simulink model "modelo_motor_P4_3"  (R2021b)
settings: Solver=VariableStepAuto  StartTime=0.0  StopTime=10.0  RelTol=1e-3
values from neighbouring files (symbols this model uses):
  Kd = Kp*Td    (= 0.032)    [lanza_P4_2.m]
  Ki = Kp/Ti    (= 11.1888111888)    [lanza_P4_2.m]
  Kp = 8    [lanza_P4_2.m]
  Tm = 0.01    [lanza_P4_1.m]    (also in lanza_P4_2.m)
settings Model: Creator=luisb  LastModifiedBy=luisb

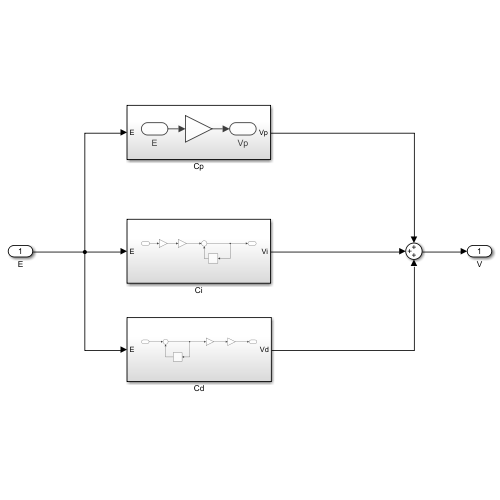
[thumbnail: Simulink's stored preview of the top-level diagram]
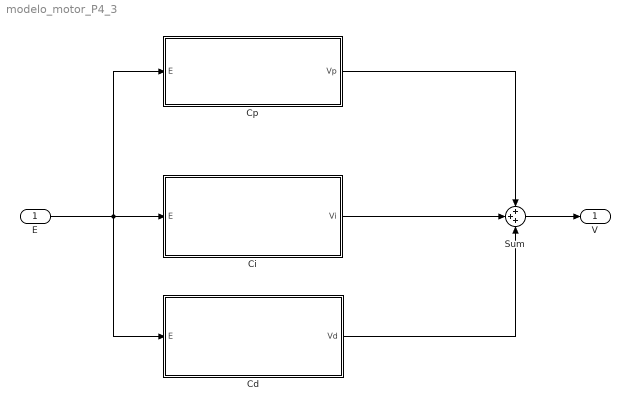
== system modelo_motor_P4_3 ==
  E : Inport
  Cd : Subsystem
  Ci : Subsystem
  Cp : Subsystem
  Sum : Sum  Inputs=+++
  V : Outport
  wires:
  Cp/1(Vp) -> Sum/1
  E/1 -> Cp/1(E), Cd/1(E), Ci/1(E)
  Ci/1(Vi) -> Sum/2
  Cd/1(Vd) -> Sum/3
  Sum/1 -> V/1

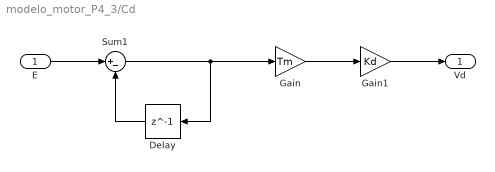
== system modelo_motor_P4_3/Cd ==
  E : Inport
  Delay : Delay  DelayLength=1  InitialCondition=0
  Gain : Gain  Gain=Tm
  Gain1 : Gain  Gain=Kd
  Sum1 : Sum  Inputs=|+-
  Vd : Outport
  wires:
  Sum1/1 -> Gain/1, Delay/1
  Delay/1 -> Sum1/2
  E/1 -> Sum1/1
  Gain/1 -> Gain1/1
  Gain1/1 -> Vd/1

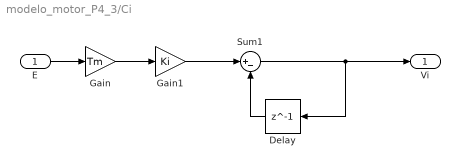
== system modelo_motor_P4_3/Ci ==
  E : Inport
  Delay : Delay  DelayLength=1  InitialCondition=0
  Gain : Gain  Gain=Tm
  Gain1 : Gain  Gain=Ki
  Sum1 : Sum  Inputs=|+-
  Vi : Outport
  wires:
  Sum1/1 -> Vi/1, Delay/1
  Gain1/1 -> Sum1/1
  Delay/1 -> Sum1/2
  Gain/1 -> Gain1/1
  E/1 -> Gain/1

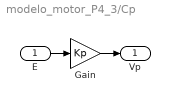
== system modelo_motor_P4_3/Cp ==
  E : Inport
  Gain : Gain  Gain=Kp
  Vp : Outport
  wires:
  Gain/1 -> Vp/1
  E/1 -> Gain/1
